simulink model "MPC_JUB27_galdir"  (R2021b)
settings: Solver=FixedStepDiscrete  StartTime=0.0  StopTime=StopTime  FixedStep=Ts  MaxStep=0.01  RelTol=1e-3
values from neighbouring files (symbols this model uses):
  dumax = [0.1 , 1]    [CarregaDados.m]    (also in Copy_of_casadi_block_Control.m = evalin('base','dumax'); casadi_block_Control.m = evalin('base','dumax'))
  f_buscaLimites_sym = evalin('base', 'f_buscaLimites_sym')    [Copy_of_casadi_block_Control.m]    (also in casadi_block_Control.m; casadi_block_Control_file.m; casadi_block_Control_galdir.m; casadi_block_Control_gov_ref.m)
  FreqAlvoIni = 55    [CarregaDados.m]
  Hc = Hp    (= 3)    [CarregaDadosMPC.m]    (also in Copy_of_casadi_block_Control.m = obj.Hc; casadi_block_Control.m = obj.Hc; casadi_block_Control_file.m = evalin('base','Hc');   obj.Hc=Hc; casadi_block_Control_galdir.m = obj.Hc)
  Hp = 3    [CarregaDadosMPC.m]    (also in Copy_of_casadi_block_Control.m = obj.Hp; casadi_block_Control.m = obj.Hp; casadi_block_Control_file.m = evalin('base','Hp');  obj.Hp=Hp; casadi_block_Control_galdir.m = obj.Hp)
  LimiteProporcao = Ts/TempoESN    (= 641.025641026)    [CarregaDados.m]
  MargemPercentual = 1    [CarregaDados.m]    (also in Copy_of_casadi_block_Control.m = evalin('base','MargemPercentual'); casadi_block_Control.m = evalin('base','MargemPercentual'))
  matriz_h = zeros(2,height(XIni))    [CarregaDados.m]    (also in Copy_of_casadi_block_Control.m = evalin('base','matriz_h'); casadi_block_Control.m = evalin('base','matriz_h'); casadi_block_Control_file.m = evalin('base','matriz_h'); casadi_block_Control_galdir.m = evalin('base','matriz_h'))
  nu = length(Qu)    [CarregaDadosMPC.m]    (also in Copy_of_casadi_block_Control.m = obj.nu; calc_ESNx_x_u.m = length(UIni); casadi_block_Control.m = obj.nu; casadi_block_Control_file.m = height(Qu))
  NumCasasDecimais = 1    [CarregaDados.m]
  nx = length(Qx)    [CarregaDadosMPC.m]    (also in Copy_of_casadi_block_Control.m = obj.nx; calc_ESN_controle.m = 10; calc_ESNx_x_u.m = height(YIni); casadi_block_Control.m = obj.nx)
  ny = length(Qy)    [CarregaDadosMPC.m]    (also in Copy_of_casadi_block_Control.m = obj.ny; casadi_block_Control.m = obj.ny; casadi_block_Control_file.m = height(Qy); casadi_block_Control_galdir.m = obj.ny)
  PassoMPC = 3    [CarregaDadosMPC.m]    (also in Copy_of_casadi_block_Control.m = obj.PassoMPC; casadi_block_Control.m = obj.PassoMPC; casadi_block_Control_file.m = evalin('base','PassoMPC'); casadi_block_Control_galdir.m = obj.PassoMPC)
  Plano = readtable('PlanoAceleracaoErro.xlsx')    [CarregaDados.m]
  PMonAlvoIni = max([PMonAlvoIni, Limites(2,2),PMonAlvoMaxMin(2)])    [CarregaDados.m]
  PMonAlvoMaxMin = [50 , 20]    [CarregaDados.m]
  Rede_Processo = load('weightsESNx_TR300_TVaz0.8_RaioE0.1.mat')    [CarregaDados.m]
  SNR = 20    [CarregaDados.m]
  Ts = 10    [CarregaDados.m]    (also in IncializaSolver.m = ModeloLSTM.temperatura_succao_BCSS.modelo_casadi.casadi_func; IncializaSolver_v2.m = ModeloLSTM.temperatura_succao_BCSS.modelo_casadi.casadi_func)
  UIni = evalin('base','UIni')    [Copy_of_casadi_block_Control.m]    (also in casadi_block_Control.m; casadi_block_Control_file.m; casadi_block_Control_galdir.m; casadi_block_Control_gov_ref.m)
  umax = [FreqMaxMin(1) ,  PMonAlvoMaxMin(1)]    [CarregaDados.m]    (also in Copy_of_casadi_block_Control.m = evalin('base','umax'); casadi_block_Control.m = evalin('base','umax'))
  umin = [FreqMaxMin(2), PMonAlvoMaxMin(2)]    [CarregaDados.m]    (also in Copy_of_casadi_block_Control.m = evalin('base','umin'); casadi_block_Control.m = evalin('base','umin'))
  UsaPlano = 0    [CarregaDados.m]
  XIni = evalin('base','XIni')    [Copy_of_casadi_block_Control.m]    (also in casadi_block_Control.m; casadi_block_Control_file.m; casadi_block_Control_galdir.m; casadi_block_Control_gov_ref.m)
undefined symbols (not defined in the file or in its folder): awgn, BTP, MatrizSimulador, MatrizSimuladorContas, TabelaIsometricas, VerHistorico
libraries: simulink x1
settings Model: Creator=odilo  LastModifiedBy=galdir
settings SolverCC: AlgebraicLoopSolver=LineSearch
settings DebuggingCC: InheritedTsInSrcMsg=none  SFMachineParentedDataDiag=warning

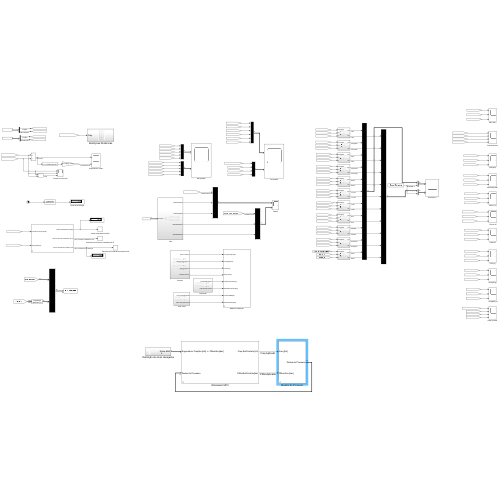
[thumbnail: Simulink's stored preview of the top-level diagram]
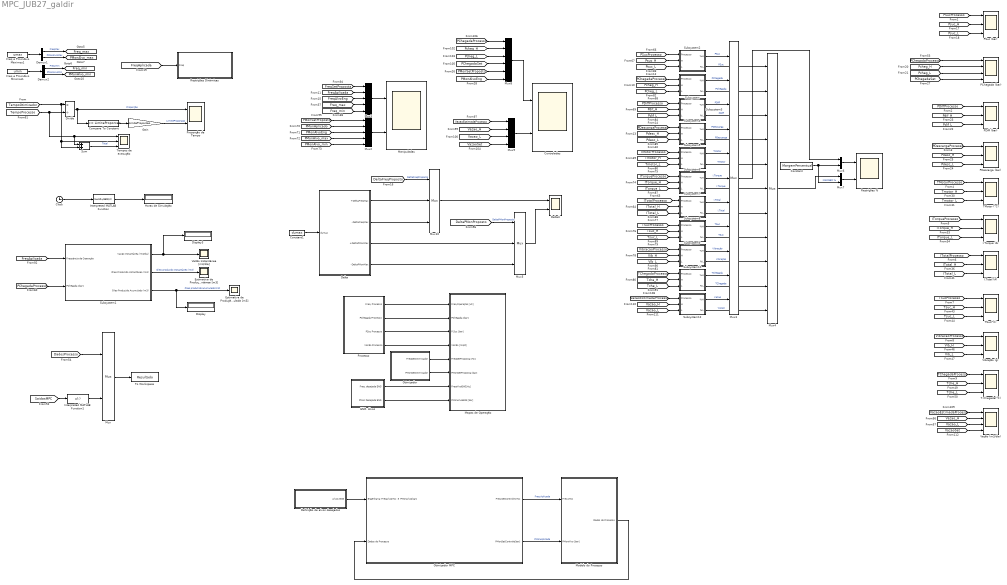
== system MPC_JUB27_galdir ==
  Clock : Clock
  Compare To Constant : simulink/Logic and Bit Operations/Compare To Constant  relop=<=  const=LimiteProporcao  OutDataTypeStr=boolean
  Constant : Constant  Value=MargemPercentual
  Constant1 : Constant  Value=dumax
  Controladas : Scope  NumInputPorts=2
  Definição de alvos desejados : Subsystem
  Delta : Subsystem
  DeltaU : Scope  NumInputPorts=2
  Demux1 : Demux  Outputs=2
  Demux2 : Demux  Outputs=2
  Display : Display
  Display3 : Display
  Divide : Product  Inputs=*/
  ENG. Alvos : Subsystem
  Estimativa de Produção Acumulada [m3] : Scope
  Estimativa de Produção instantânea [m3] : Scope
  Freq e PmonAlvo Máximos1 : Constant  Value=umax
  Freq e PmonAlvo Mínimos1 : Constant  Value=umin
  Gain : Gain  Gain=LimiteProporcao
  Horas de Simulação : Display
  I.Torque (A) : Scope  NumInputPorts=3
  I.Total (A) : Scope  NumInputPorts=3
  Interpreted MATLAB Function : MATLABFcn  MATLABFcn=round(u/3600,2)
  Interpreted MATLAB Function1 : MATLABFcn  MATLABFcn=u(:)
  Manipuladas : Scope  NumInputPorts=2
  Mapas de Operação : Subsystem  mask{PlotaMapas=1, HabilitaRastro=1, MatrizSimulador=MatrizSimulador, MatrizSimuladorContas=MatrizSimuladorContas, BTP=BTP, TabelaIsometricas=TabelaIsometricas, FreqIni=UIni(1), PChegadaIni=XIni(2), PSucIni=XIni(1), VazaoIni=XIni(11), MargemPercentual=MargemPercentual, FreqAlvoIni=FreqAlvoIni, PMonAlvoIni=PMonAlvoIni, PMonAlvoMaxMin=PMonAlvoMaxMin}
      mask prompts: PlotaMapas "Plotar Mapas (1/0)?"; HabilitaRastro "Habilita Rastro do Plot (1/0)?"; MatrizSimulador "Matriz do Simulador"; MatrizSimuladorContas "Matriz do Simulador para Limites"; BTP "Matriz BTP"; TabelaIsometricas "Tabela Curvas Isometricas"; FreqIni "Frequencia Inicial [Hz]"; PChegadaIni "PChegada Inicial [bar]"; PSucIni "PSuc Inicial [bar]"; VazaoIni "Vazao Inicial [m3/d]"; MargemPercentual "Margem % de folga para os alarmes"; FreqAlvoIni "Frequencia ALVO Inicial [Hz]"; PMonAlvoIni "PChegada ALVO [bar]"; PMonAlvoMaxMin "PMonAlvo [Max  Min]"
      mask DialogControl DescTextVar Prompt: MAPAS DE OPERAÇÃO
      mask DialogControl ParameterGroupVar Prompt: Tabelas Petrobras e configurações dos Mapas de Operação
      mask DialogControl ParameterGroupVar_copy Prompt: Dados do Processo
      mask DialogControl ParameterGroupVar_copy_copy_copy Prompt: Dados Engenharia (Alvos)
  Modelo do Processo : Subsystem  mask{ESN=Rede_Processo, YIni=XIni, UIni=UIni, SNR=SNR, NumCasasDecimais=NumCasasDecimais, MatrizSimulador=MatrizSimulador}
      mask prompts: ESN "Estruturada ESN"; YIni "Condicoes iniciais das variaveis"; UIni "Condicao Inicial das manipuladas (Freq e PMon)"; SNR "Relação Sinal Ruido aplicada"; NumCasasDecimais "Numero de casas decimais"; MatrizSimulador "Matriz do Simulador Petrobras"
  Mux : Mux  Inputs=2
  Mux1 : Mux  Inputs=5
  Mux10 : Mux  Inputs=3
  Mux2 : Mux  Inputs=5
  Mux3 : Mux  Inputs=11
  Mux4 : Mux  Inputs=11
  Mux5 : Mux  Inputs=3
  Mux6 : Mux  Inputs=2
  Mux7 : Mux  Inputs=2
  Mux8 : Mux  Inputs=6
  Mux9 : Mux
  Otimizador : Subsystem
  Otimizador MPC : Subsystem  mask{Hp=Hp, Hc=Hc, PassoMPC=PassoMPC, nx=nx, ny=ny, nu=nu}
      mask prompts: Hp "Horizonte de Predicao"; Hc "Horizonte de Controle"; PassoMPC "Passos para o controle atuar"; nx "Numero de Estados X"; ny "Numero de Saidas Y (controladas por setpoint)"; nu "Numero de entradas (acoes de controle)"
      mask DialogControl ControlParameters Prompt: PARAMETROS DO CONTROLADOR
      mask DialogControl SaidasCasadi Prompt: DIMENSIONAR SAIDAS CasadiBlock
  PChegada (bar) : Scope  NumInputPorts=4
  PDescarga (bar) : Scope  NumInputPorts=3
  PDiff (bar) : Scope  NumInputPorts=3
  PSuc (bar) : Scope  NumInputPorts=3
  Processo : Subsystem
  Proporção de Tempo : Scope  NumInputPorts=2
  Restrições % : Scope  NumInputPorts=2
  Restrições Dinâmicas : Subsystem
  Subsystem : Subsystem
  Subsystem1 : Subsystem  mask{MatrizSimulador=MatrizSimulador, DeltaT=Ts, QIni=XIni(11)}
      mask prompts: MatrizSimulador "Matriz do Simulador Petrobras"; DeltaT "Periodo de amostragem (s)"; QIni "Vazao Inicial (m3/dia)"
  Subsystem10 : Subsystem
  Subsystem12 : Subsystem
  Subsystem2 : Subsystem
  Subsystem3 : Subsystem
  Subsystem4 : Subsystem
  Subsystem5 : Subsystem
  Subsystem6 : Subsystem
  Subsystem7 : Subsystem
  Subsystem8 : Subsystem
  Subsystem9 : Subsystem
  Sum : Sum
  T.Chegada(°C) : Scope  NumInputPorts=3
  TMotor (°C) : Scope  NumInputPorts=3
  TSuc(°C) : Scope  NumInputPorts=3
  Tempos de execução : Scope  NumInputPorts=3
  To Workspace : ToWorkspace  VariableName=Resultado  SampleTime=-1
  Vazão (m3/dia) : Scope  NumInputPorts=4
  Vazão Instantânea [m3/dia] : Scope
  Vibração (g) : Scope  NumInputPorts=3
  tag scope: Freq_max=global, Freq_min=global, PMonAlvo_max=global, PMonAlvo_min=global
  wires:
  [TempoProcesso] -> Sum/1, Tempos de execução/1, Divide/2
  [ITotalProcesso] -> I.Total (A)/1
  [TMotorProcesso] -> TMotor (°C)/1
  [VibracaoProcesso] -> Vibração (g)/1
  [TSucProcesso] -> TSuc(°C)/1
  [PDiffProcesso] -> PDiff (bar)/1
  [PDescargaProcesso] -> PDescarga (bar)/1
  [PSucProcesso] -> PSuc (bar)/1
  [Freq_max] -> Mux1/4
  [Freq_min] -> Mux1/5
  [FreqAlvoEng] -> Mux1/3
  [Psuc_H] -> PSuc (bar)/2
  [Psuc_L] -> PSuc (bar)/3
  [Pdif_H] -> PDiff (bar)/2
  [Pdif_L] -> PDiff (bar)/3
  [Pdesc_H] -> PDescarga (bar)/2
  [Pdesc_L] -> PDescarga (bar)/3
  [Tmotor_H] -> TMotor (°C)/2
  [Tmotor_L] -> TMotor (°C)/3
  [ITorqueProcesso] -> I.Torque (A)/1
  [ITorque_H] -> I.Torque (A)/2
  [ITorque_L] -> I.Torque (A)/3
  [ITotal_H] -> I.Total (A)/2
  [ITotal_L] -> I.Total (A)/3
  [Tsuc_H] -> TSuc(°C)/2
  [Tsuc_L] -> TSuc(°C)/3
  [Vib_H] -> Vibração (g)/2
  [Vib_L] -> Vibração (g)/3
  [TChegadaProcesso] -> T.Chegada(°C)/1
  [Tche_H] -> T.Chegada(°C)/2
  [Tche_L] -> T.Chegada(°C)/3
  Mux/1 -> To Workspace/1
  [DadosProcesso] -> Mux/1
  [FreqAplicada] -> Mux1/2
  [PChegadaProcesso] -> PChegada (bar)/1
  [Pcheg_H] -> PChegada (bar)/2
  [Pcheg_L] -> PChegada (bar)/3
  [PChegadaSet] -> PChegada (bar)/4
  [TempoOtimizador] -> Sum/2, Tempos de execução/2, Divide/1
  [FreqAplicada] -> Subsystem1/1(Frequência de Operação)
  [PChegadaProcesso] -> Subsystem1/2(PChegada [bar])
  Subsystem1/2("Óleo Produzido Instantâneo (m3) ") -> Estimativa de Produção instantânea [m3]/1  "Óleo produzido Instantâneo (m3)"
  Subsystem1/3(Óleo Produzido Acumulado (m3)) -> Display/1, Estimativa de Produção Acumulada [m3]/1  "Óleo produzido acumulado(m3)"
  Subsystem1/1(Vazão Instantânea (m3/dia)) -> Display3/1, Vazão Instantânea [m3/dia]/1
  Sum/1 -> Tempos de execução/3  "Total"
  Mux1/1 -> Manipuladas/1
  [PMonAlvo_min] -> Mux2/5
  [PMonAlvo_max] -> Mux2/4
  [PMonAplicado] -> Mux2/2
  Mux2/1 -> Manipuladas/2
  [PChegadaProcesso] -> Subsystem/1(Processo)
  [Pcheg_H] -> Subsystem/2(H)
  [Pcheg_L] -> Subsystem/3(L)
  [PSucProcesso] -> Subsystem2/1(Processo)
  [Psuc_H] -> Subsystem2/2(H)
  [Psuc_L] -> Subsystem2/3(L)
  [PDiffProcesso] -> Subsystem3/1(Processo)
  [Pdif_H] -> Subsystem3/2(H)
  [Pdif_L] -> Subsystem3/3(L)
  [PDescargaProcesso] -> Subsystem4/1(Processo)
  [Pdesc_H] -> Subsystem4/2(H)
  [Pdesc_L] -> Subsystem4/3(L)
  [Tmotor_L] -> Subsystem5/3(L)
  [Tmotor_H] -> Subsystem5/2(H)
  [TMotorProcesso] -> Subsystem5/1(Processo)
  [ITorqueProcesso] -> Subsystem6/1(Processo)
  [ITorque_H] -> Subsystem6/2(H)
  [ITorque_L] -> Subsystem6/3(L)
  [ITotalProcesso] -> Subsystem7/1(Processo)
  [ITotal_H] -> Subsystem7/2(H)
  [ITotal_L] -> Subsystem7/3(L)
  [TSucProcesso] -> Subsystem8/1(Processo)
  [Tsuc_H] -> Subsystem8/2(H)
  [Tsuc_L] -> Subsystem8/3(L)
  [VibracaoProcesso] -> Subsystem9/1(Processo)
  [Vib_H] -> Subsystem9/2(H)
  [Vib_L] -> Subsystem9/3(L)
  [TChegadaProcesso] -> Subsystem10/1(Processo)
  [Tche_H] -> Subsystem10/2(H)
  [Tche_L] -> Subsystem10/3(L)
  Mux3/1 -> Mux6/1
  Mux4/1 -> Mux7/1
  Subsystem/2(%L) -> Mux4/2  "PChegada"
  Subsystem2/2(%L) -> Mux4/1  "PSuc"
  Subsystem/1(%H) -> Mux3/2  "PChegada"
  Subsystem2/1(%H) -> Mux3/1  "PSuc"
  Subsystem3/1(%H) -> Mux3/3  "PDiff"
  Subsystem3/2(%L) -> Mux4/3  "PDiff"
  Subsystem4/1(%H) -> Mux3/4  "PDescarga"
  Subsystem4/2(%L) -> Mux4/4  "PDescarga"
  Subsystem5/2(%L) -> Mux4/5  "TMotor"
  Subsystem5/1(%H) -> Mux3/5  "TMotor"
  Subsystem6/2(%L) -> Mux4/6  "I.Torque"
  Subsystem6/1(%H) -> Mux3/6  "I.Torque"
  Subsystem7/2(%L) -> Mux4/7  "I.Total"
  Subsystem7/1(%H) -> Mux3/7  "I.Total"
  Subsystem8/2(%L) -> Mux4/8  "TSuc"
  Subsystem8/1(%H) -> Mux3/8  "TSuc"
  Subsystem9/2(%L) -> Mux4/9  "Vibração"
  Mux10/1 -> DeltaU/1
  Constant1/1 -> Delta/1(dumax)
  Delta/2(-DeltaFreqMax) -> Mux10/3
  Clock/1 -> Interpreted MATLAB Function/1
  Interpreted MATLAB Function/1 -> Horas de Simulação/1
  [DeltaPMonProposto] -> Mux5/1  "DeltaPMonProposto"
  Delta/3(+DeltaPMonMax) -> Mux5/2
  Delta/4(-DeltaPMonMax) -> Mux5/3
  [PChegadaSet] -> Mux8/4
  [Pcheg_L] -> Mux8/3
  [Pcheg_H] -> Mux8/2
  [PChegadaProcesso] -> Mux8/1
  [VazaoSet] -> Mux9/4
  [Vazao_L] -> Mux9/3
  [Vazao_H] -> Mux9/2
  [VazaoEstimadaProcesso] -> Mux9/1
  Mux9/1 -> Controladas/2
  Mux8/1 -> Controladas/1
  Processo/1(Freq. Processo) -> Mapas de Operação/1(Freq.Operação [Hz])
  Processo/2(PChegada Processo) -> Mapas de Operação/2(PChegada [bar])
  ENG. Alvos/1(Freq. desejada ENG) -> Mapas de Operação/7(FreqAlvoENG[Hz])
  ENG. Alvos/2(PMon Desejada ENG) -> Mapas de Operação/8(PMonAlvoENG [bar])
  Processo/3(PSuc Processo) -> Mapas de Operação/3(P.Suc [bar])
  Delta/1(+DeltaFreqMax) -> Mux10/2
  Otimizador MPC/1(Freq.SetControle [Hz]) -> Modelo do Processo/1(Freq [Hz])  "Freq.Aplicada"
  Otimizador MPC/2(PMonSetControle[bar]) -> Modelo do Processo/2(PMonAlvo [bar])  "PMonAplicada"
  [FreqSetProposta] -> Mux1/1
  [PMonSetProposto] -> Mux2/1
  [PMonAlvoEng] -> Mux2/3
  [Vazao_L] -> Vazão (m3/dia)/3
  [Vazao_H] -> Vazão (m3/dia)/2
  [VazaoEstimadaProcesso] -> Vazão (m3/dia)/1
  [VazaoEstimadaProcesso] -> Subsystem12/1(Processo)
  [Vazao_H] -> Subsystem12/2(H)
  [Vazao_L] -> Subsystem12/3(L)
  Subsystem12/1(%H) -> Mux3/11  "Vazao"
  Subsystem12/2(%L) -> Mux4/11  "Vazao"
  Subsystem10/2(%L) -> Mux4/10  "TChegada"
  Subsystem9/1(%H) -> Mux3/9  "Vibração"
  Subsystem10/1(%H) -> Mux3/10  "TChegada"
  [VazaoSet] -> Vazão (m3/dia)/4
  Modelo do Processo/1(Dados do Processo) -> Otimizador MPC/2(Dados do Processo)
  Divide/1 -> Proporção de Tempo/1, Compare To Constant/1  "Proporção"
  Compare To Constant/1 -> Gain/1
  Gain/1 -> Proporção de Tempo/2  "LimiteProporção"
  Definição de alvos desejados/1(Alvos ENG) -> Otimizador MPC/1(Engenharia: FreqAlvo[Hz]  e  PMonAlvo[bar])
  Demux1/1 -> [Freq_max]  "FreqMax"
  Demux2/1 -> [Freq_min]  "Freq.Min"
  Demux1/2 -> [PMonAlvo_max]  "PMonAlvoMax"
  Demux2/2 -> [PMonAlvo_min]  "PMonAlvoMin"
  Freq e PmonAlvo Mínimos1/1 -> Demux2/1
  Freq e PmonAlvo Máximos1/1 -> Demux1/1
  [FreqAplicada] -> Restrições Dinâmicas/1(Freq)
  Processo/4(Vazão Processo) -> Mapas de Operação/4(Vazão [m3/d])
  Otimizador/1(FreqSetOtimizador) -> Mapas de Operação/5(FreqSetProposta [Hz])
  Otimizador/2(PMonSetOtimizador) -> Mapas de Operação/6(PMonSetProposta [bar])
  [DeltaFreqProposto] -> Mux10/1  "DeltaFreqProposto"
  Mux5/1 -> DeltaU/2
  [PMonSetProposto] -> Mux8/5
  [PMonAlvoEng] -> Mux8/6
  Mux6/1 -> Restrições %/1
  Constant/1 -> Mux6/2, Mux7/2  "MARGEM %"
  Mux7/1 -> Restrições %/2
  [SaidasMPC] -> Interpreted MATLAB Function1/1
  Interpreted MATLAB Function1/1 -> Mux/2

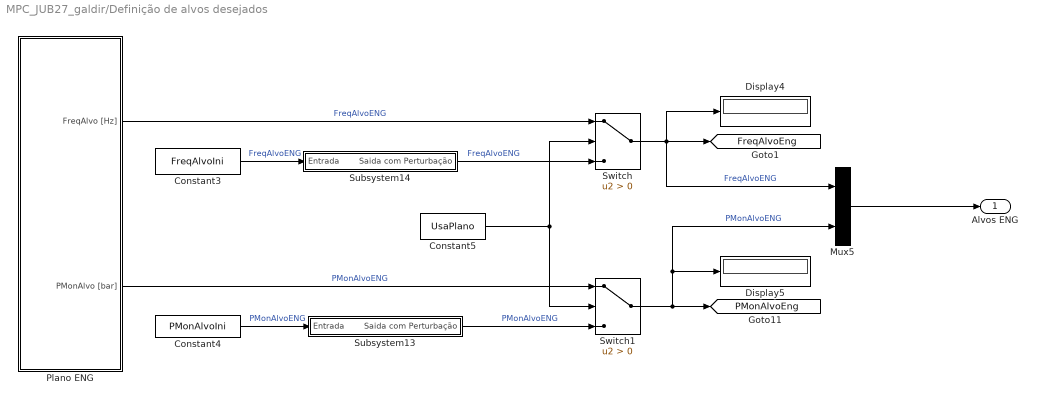
== system MPC_JUB27_galdir/Definição de alvos desejados ==
  Constant3 : Constant  Value=FreqAlvoIni
  Constant4 : Constant  Value=PMonAlvoIni
  Constant5 : Constant  Value=UsaPlano
  Display4 : Display
  Display5 : Display
  Mux5 : Mux  Inputs=2
  Plano ENG : Subsystem  mask{Plano=Plano}
      mask prompts: Plano "Plano de Execucao"
      mask DialogControl DescGroupVar Prompt: TABELA COM PLANO DE EXECUCAO
  Subsystem13 : Subsystem  mask{TIni=1200, DeltaT=1.5*3600, ValorP=0}
      mask prompts: TIni "Tempo Inicio"; DeltaT "Duracao"; ValorP "Valor da Perturbacao"
  Subsystem14 : Subsystem  mask{TIni=1200, DeltaT=1.5*3600, ValorP=0}
      mask prompts: TIni "Tempo Inicio"; DeltaT "Duracao"; ValorP "Valor da Perturbacao"
  Switch : Switch  Criteria=u2 > Threshold
  Switch1 : Switch  Criteria=u2 > Threshold
  Alvos ENG : Outport
  tag scope: FreqAlvoEng=global, PMonAlvoEng=global
  wires:
  Constant5/1 -> Switch1/2, Switch/2
  Subsystem14/1(Saida com Perturbação) -> Switch/3  "FreqAlvoENG"
  Constant3/1 -> Subsystem14/1(Entrada)  "FreqAlvoENG"
  Switch/1 -> Mux5/1, [FreqAlvoEng], Display4/1  "FreqAlvoENG"
  Switch1/1 -> Mux5/2, Display5/1, [PMonAlvoEng]  "PMonAlvoENG"
  Plano ENG/1(FreqAlvo [Hz]) -> Switch/1  "FreqAlvoENG"
  Subsystem13/1(Saida com Perturbação) -> Switch1/3  "PMonAlvoENG"
  Plano ENG/2(PMonAlvo [bar]) -> Switch1/1  "PMonAlvoENG"
  Constant4/1 -> Subsystem13/1(Entrada)  "PMonAlvoENG"
  Mux5/1 -> Alvos ENG/1

== system MPC_JUB27_galdir/Delta ==
  dumax : Inport
  Demux : Demux  Outputs=2
  Gain : Gain  Gain=-1
  Gain6 : Gain  Gain=-1
  +DeltaFreqMax : Outport
  -DeltaFreqMax : Outport  Port=2
  +DeltaPMonMax : Outport  Port=3
  -DeltaPMonMax : Outport  Port=4
  wires:
  Demux/1 -> Gain/1, +DeltaFreqMax/1  "+DeltaFreqMax"
  Demux/2 -> Gain6/1, +DeltaPMonMax/1  "+DeltaPMonMax"
  dumax/1 -> Demux/1
  Gain/1 -> -DeltaFreqMax/1  "-DeltaFreqMax"
  Gain6/1 -> -DeltaPMonMax/1  "-DeltaPMonMax"

== system MPC_JUB27_galdir/ENG. Alvos ==
  Freq. desejada ENG : Outport
  PMon Desejada ENG : Outport  Port=2
  wires:
  [PMonAlvoEng] -> PMon Desejada ENG/1
  [FreqAlvoEng] -> Freq. desejada ENG/1

== system MPC_JUB27_galdir/Mapas de Operação ==
  Freq.Operação [Hz] : Inport
  PChegada [bar] : Inport  Port=2
  P.Suc [bar] : Inport  Port=3
  Vazão [m3/d] : Inport  Port=4
  FreqSetProposta [Hz] : Inport  Port=5
  PMonSetProposta [bar] : Inport  Port=6
  FreqAlvoENG[Hz] : Inport  Port=7
  PMonAlvoENG [bar] : Inport  Port=8
  Mux : Mux  Inputs=8
  S-Function : S-Function  FunctionName=AnimaMapa  Parameters=PlotaMapas,MatrizSimulador,MatrizSimuladorContas,BTP,FreqIni, PChegadaIni,PSucIni,VazaoIni,FreqAlvoIni,PMonAlvoIni,HabilitaRastro,TabelaIsometricas,MargemPercentual,PMonAlvoMaxMin  SFunctionDeploymentMode=off  EnableBusSupport=off
  wires:
  FreqSetProposta [Hz]/1 -> Mux/5
  PMonAlvoENG [bar]/1 -> Mux/8
  FreqAlvoENG[Hz]/1 -> Mux/7
  PMonSetProposta [bar]/1 -> Mux/6
  Vazão [m3/d]/1 -> Mux/4
  PChegada [bar]/1 -> Mux/2
  Mux/1 -> S-Function/1
  Freq.Operação [Hz]/1 -> Mux/1
  P.Suc [bar]/1 -> Mux/3

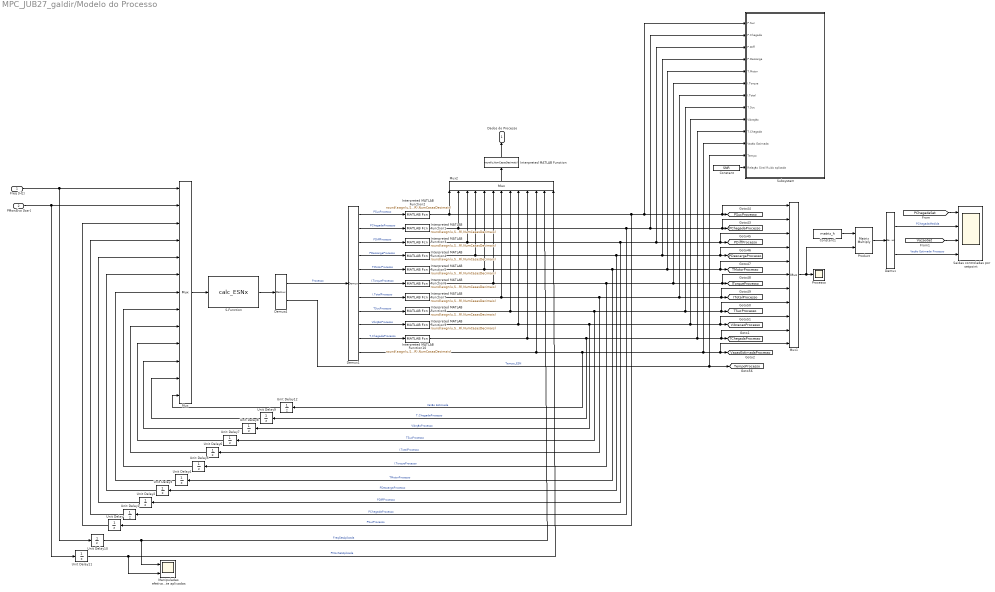
== system MPC_JUB27_galdir/Modelo do Processo ==
  Freq [Hz] : Inport
  PMonAlvo [bar] : Inport  Port=2
  Constant : Constant  Value=SNR
  Constant1 : Constant  Value=matriz_h
  Demux : Demux  Outputs=2
  Demux1 : Demux  Outputs=11
  Demux4 : Demux  Outputs=[ 11 1]
  Interpreted MATLAB Function : MATLABFcn  MATLABFcn=round(u,NumCasasDecimais)
  Interpreted MATLAB Function{1..10} (10 alike) : MATLABFcn  MATLABFcn=round(awgn(u,SNR),NumCasasDecimais)
  Manipuladas efetivamente aplicadas : Scope  NumInputPorts=2
  Mux : Mux  Inputs=2+11
  Mux1 : Mux  Inputs=11
  Mux2 : Mux  Inputs=13
  Processo : Scope
  Product : Product  Multiplication=Matrix(*)
  S-Function : S-Function  FunctionName=calc_ESNx  Parameters=ESN.data,YIni,MatrizSimulador  SFunctionDeploymentMode=off  EnableBusSupport=off
  Saidas controladas por setpoint : Scope  NumInputPorts=4
  Subsystem : Subsystem
  Unit Delay : UnitDelay  InitialCondition=YIni(1)  SampleTime=-1  HasFrameUpgradeWarning=on
  Unit Delay1 : UnitDelay  InitialCondition=YIni(2)  SampleTime=-1  HasFrameUpgradeWarning=on
  Unit Delay10 : UnitDelay  InitialCondition=UIni(1)  SampleTime=-1  HasFrameUpgradeWarning=on
  Unit Delay11 : UnitDelay  InitialCondition=UIni(2)  SampleTime=-1  HasFrameUpgradeWarning=on
  Unit Delay12 : UnitDelay  InitialCondition=YIni(11)  SampleTime=-1  HasFrameUpgradeWarning=on
  Unit Delay2 : UnitDelay  InitialCondition=YIni(3)  SampleTime=-1  HasFrameUpgradeWarning=on
  Unit Delay3 : UnitDelay  InitialCondition=YIni(4)  SampleTime=-1  HasFrameUpgradeWarning=on
  Unit Delay4 : UnitDelay  InitialCondition=YIni(5)  SampleTime=-1  HasFrameUpgradeWarning=on
  Unit Delay5 : UnitDelay  InitialCondition=YIni(6)  SampleTime=-1  HasFrameUpgradeWarning=on
  Unit Delay6 : UnitDelay  InitialCondition=YIni(7)  SampleTime=-1  HasFrameUpgradeWarning=on
  Unit Delay7 : UnitDelay  InitialCondition=YIni(8)  SampleTime=-1  HasFrameUpgradeWarning=on
  Unit Delay8 : UnitDelay  InitialCondition=YIni(9)  SampleTime=-1  HasFrameUpgradeWarning=on
  Unit Delay9 : UnitDelay  InitialCondition=YIni(10)  SampleTime=-1  HasFrameUpgradeWarning=on
  Dados do Processo : Outport
  tag scope: ITorqueProcesso=global, ITotalProcesso=global, PChegadaProcesso=global, PDescargaProcesso=global, PDiffProcesso=global, PSucProcesso=global, TChegadaProcesso=global, TMotorProcesso=global, TSucProcesso=global, TempoProcesso=global, VazaoEstimadaProcesso=global, VibracaoProcesso=global
  wires:
  Mux/1 -> S-Function/1
  PMonAlvo [bar]/1 -> Unit Delay11/1, Mux/2
  Freq [Hz]/1 -> Unit Delay10/1, Mux/1
  Unit Delay/1 -> Mux/3
  Unit Delay1/1 -> Mux/4
  Unit Delay2/1 -> Mux/5
  Unit Delay3/1 -> Mux/6
  Unit Delay4/1 -> Mux/7
  Unit Delay5/1 -> Mux/8
  Unit Delay6/1 -> Mux/9
  Unit Delay7/1 -> Mux/10
  Unit Delay8/1 -> Mux/11
  Unit Delay9/1 -> Mux/12
  S-Function/1 -> Demux4/1
  Demux1/4 -> Interpreted MATLAB Function4/1  "PDescargaProcesso"
  Demux1/3 -> Interpreted MATLAB Function3/1  "PDiffProcesso"
  Demux1/9 -> Interpreted MATLAB Function9/1  "VibrçãoProcesso"
  Demux1/7 -> Interpreted MATLAB Function7/1  "I.TotalProcesso"
  Demux1/10 -> Interpreted MATLAB Function10/1  "T,ChegadaProcesso"
  Demux4/2 -> Subsystem/12(Tempo), [TempoProcesso]  "Tempo_ESN"
  Interpreted MATLAB Function2/1 -> Unit Delay/1, Subsystem/1(P.Suc), Mux1/1, [PSucProcesso], Mux2/1  "PSucProcesso"
  Interpreted MATLAB Function1/1 -> Subsystem/2(P.Chegada), Mux1/2, [PChegadaProcesso], Unit Delay1/1, Mux2/2  "PChegadaProcesso"
  Interpreted MATLAB Function3/1 -> Subsystem/3(P.Diff), Mux1/3, [PDiffProcesso], Unit Delay2/1, Mux2/3  "PDiffProcesso"
  Interpreted MATLAB Function4/1 -> Subsystem/4(P.Descarga), Mux1/4, [PDescargaProcesso], Unit Delay3/1, Mux2/4  "PDescargaProcesso"
  Interpreted MATLAB Function5/1 -> Subsystem/5(T.Motor), Mux1/5, [TMotorProcesso], Unit Delay4/1, Mux2/5  "TMotorProcesso"
  Interpreted MATLAB Function6/1 -> Subsystem/6(I.Torque), Mux1/6, [ITorqueProcesso], Unit Delay5/1, Mux2/6  "I.TorqueProcesso"
  Interpreted MATLAB Function7/1 -> Subsystem/7(I.Total), Mux1/7, [ITotalProcesso], Unit Delay6/1, Mux2/7  "I.TotalProcesso"
  Interpreted MATLAB Function8/1 -> Subsystem/8(T.Suc), Mux1/8, [TSucProcesso], Unit Delay7/1, Mux2/8  "TSucProcesso"
  Interpreted MATLAB Function9/1 -> Subsystem/9(Vibração), Mux1/9, [VibracaoProcesso], Unit Delay8/1, Mux2/9  "VibrçãoProcesso"
  Interpreted MATLAB Function10/1 -> Unit Delay9/1, Mux1/10, [TChegadaProcesso], Subsystem/10(T.Chegada), Mux2/10  "T,ChegadaProcesso"
  Constant/1 -> Subsystem/13(Relação Sinal Ruido aplicada)
  Demux1/1 -> Interpreted MATLAB Function2/1  "PSucProcesso"
  Demux1/2 -> Interpreted MATLAB Function1/1  "PChegadaProcesso"
  Demux1/5 -> Interpreted MATLAB Function5/1  "TMotorProcesso"
  Demux1/6 -> Interpreted MATLAB Function6/1  "I.TorqueProcesso"
  Demux1/8 -> Interpreted MATLAB Function8/1  "TSucProcesso"
  Interpreted MATLAB Function/1 -> Dados do Processo/1
  Demux4/1 -> Demux1/1  "Processo"
  Unit Delay10/1 -> Mux2/12, Manipuladas efetivamente aplicadas/1  "FreqSetAplicada"
  Unit Delay11/1 -> Mux2/13, Manipuladas efetivamente aplicadas/2  "PMonSetAplicada"
  Demux1/11 -> Subsystem/11(Vazão Estimada), Mux1/11, [VazaoEstimadaProcesso], Unit Delay12/1, Mux2/11  "Vazão Estimada"
  Unit Delay12/1 -> Mux/13
  Product/1 -> Demux/1
  Constant1/1 -> Product/1
  Mux1/1 -> Product/2, Processo/1
  [PChegadaSet] -> Saidas controladas por setpoint/1
  [VazaoSet] -> Saidas controladas por setpoint/3
  Demux/1 -> Saidas controladas por setpoint/2  "PChegadaMedida"
  Demux/2 -> Saidas controladas por setpoint/4  "Vazão Estimada Processo"
  Mux2/1 -> Interpreted MATLAB Function/1

== system MPC_JUB27_galdir/Otimizador ==
  FreqSetOtimizador : Outport
  PMonSetOtimizador : Outport  Port=2
  wires:
  [FreqSetProposta] -> FreqSetOtimizador/1
  [PMonSetProposto] -> PMonSetOtimizador/1

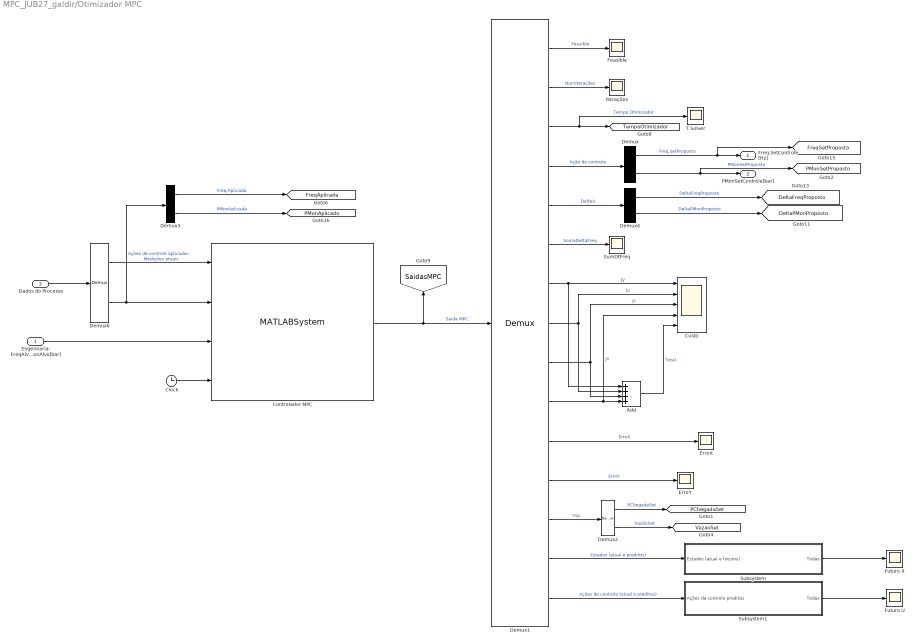
== system MPC_JUB27_galdir/Otimizador MPC ==
  Engenharia: FreqAlvo[Hz]  e  PMonAlvo[bar] : Inport
  Dados do Processo : Inport  Port=2
  Add : Sum  Inputs=++++
  Clock : Clock
  Controlador MPC : MATLABSystem  System=casadi_block_Control  SimulateUsing=Interpreted execution
      mask Type: casadi_block_Control
      mask Display:
      | disp('casadi_block_Control');
      | port_label('input',1,'X0');
      | port_label('input',2,'U0');
      | port_label('input',3,'AlvoEng');
      | port_label('input',4,'t');
      | port_label('output',1,'SaidaMPC');
  "Custo " : Scope  NumInputPorts=5
  Demux{,2..4} (4 alike) : Demux  Outputs=2
  Demux1 : Demux  Outputs="[ 1  1  1  nu  nu  1  1  1  1  1  nx  ny  ny    nx+nx*Hp   nu*Hp ]"
  Demux6 : Demux  Outputs=[11 2]
  ErroX : Scope
  ErroY : Scope
  Feasible : Scope
  Futuro U : Scope
  Futuro X : Scope
  Iterações : Scope
  Subsystem : Subsystem
  Subsystem1 : Subsystem
  SumDtFreq : Scope
  T.Solver : Scope
  Freq.SetControle [Hz] : Outport
  PMonSetControle[bar] : Outport  Port=2
  tag scope: DeltaFreqProposto=global, DeltaPMonProposto=global, FreqAplicada=global, FreqSetProposta=global, PChegadaSet=global, PMonAplicado=global, PMonSetProposto=global, SaidasMPC=global, TempoOtimizador=global, VazaoSet=global
  wires:
  Demux1/3 -> T.Solver/1, [TempoOtimizador]  "Tempo Otimizador"
  Demux1/1 -> Feasible/1  "Feasible"
  Demux4/1 -> [DeltaFreqProposto]  "DeltaFreqProposto"
  Demux/1 -> [FreqSetProposta], Freq.SetControle [Hz]/1  "Freq.SetProposto"
  Demux/2 -> [PMonSetProposto], PMonSetControle[bar]/1  "PMonSetProposto"
  Demux4/2 -> [DeltaPMonProposto]  "DeltaPMonProposto"
  Dados do Processo/1 -> Demux6/1
  Demux6/1 -> Controlador MPC/1  "Medições atuais"
  Demux6/2 -> Demux3/1, Controlador MPC/2  "Ações de controle aplicadas"
  Demux1/4 -> Demux/1  "Ação de controle"
  Demux1/2 -> Iterações/1  "NumIterações"
  Demux1/5 -> Demux4/1  "DeltaU"
  Controlador MPC/1 -> [SaidasMPC], Demux1/1  "Saida MPC"
  Demux2/1 -> [PChegadaSet]  "PChegadaSet"
  Engenharia: FreqAlvo[Hz]  e  PMonAlvo[bar]/1 -> Controlador MPC/3
  Demux2/2 -> [VazaoSet]  "VazãoSet"
  Clock/1 -> Controlador MPC/4
  Demux3/2 -> [PMonAplicado]  "PMonAplicada"
  Demux3/1 -> [FreqAplicada]  "Freq.Aplicada"
  Demux1/14 -> Subsystem/1(Estados (atual e futuros))  "Estados (atual e preditos)"
  Subsystem/1(Todas) -> Futuro X/1
  Subsystem1/1(Todas) -> Futuro U/1
  Demux1/6 -> SumDtFreq/1  "SomaDeltaFreq"
  Demux1/7 -> "Custo "/1, Add/1  "Jy"
  Demux1/8 -> "Custo "/2, Add/2  "Ju"
  Demux1/9 -> "Custo "/3, Add/3  "Jr"
  Demux1/13 -> Demux2/1  "Ysp"
  Demux1/10 -> "Custo "/4, Add/4  "Jx"
  Add/1 -> "Custo "/5  "Total"
  Demux1/15 -> Subsystem1/1(Ações de controle preditas)  "Ações de controle (atual e preditos)"
  Demux1/11 -> ErroX/1  "ErroX"
  Demux1/12 -> ErroY/1  "ErroY"

== system MPC_JUB27_galdir/Processo ==
  Freq. Processo : Outport
  PChegada Processo : Outport  Port=2
  PSuc Processo : Outport  Port=3
  Vazão Processo : Outport  Port=4
  wires:
  [PSucProcesso] -> PSuc Processo/1
  [FreqAplicada] -> Freq. Processo/1
  [PChegadaProcesso] -> PChegada Processo/1
  [VazaoEstimadaProcesso] -> Vazão Processo/1

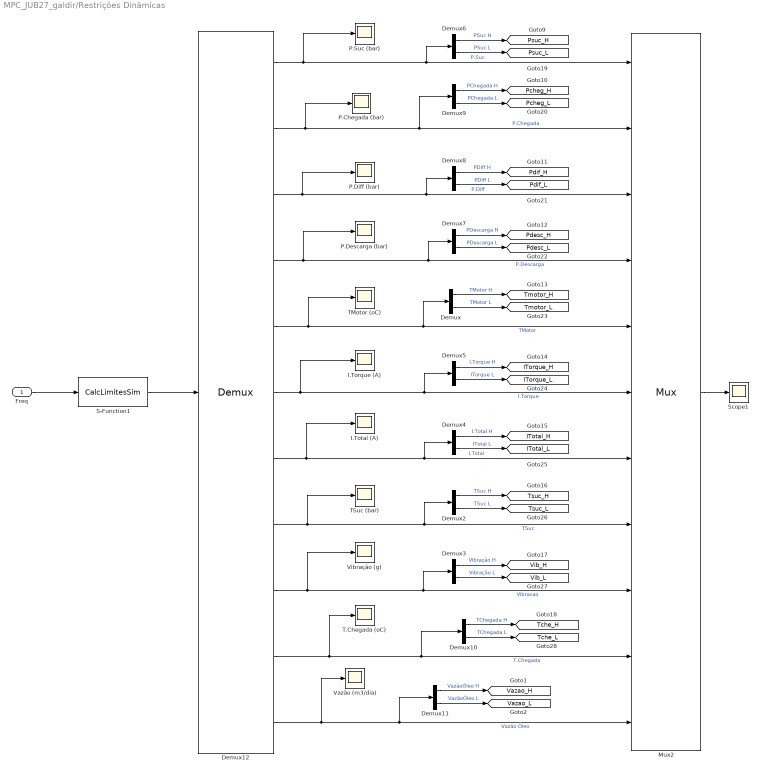
== system MPC_JUB27_galdir/Restrições Dinâmicas ==
  Freq : Inport
  Demux{,2..11} (11 alike) : Demux  Outputs=2
  Demux12 : Demux  Outputs=[ 2 2 2 2 2 2 2 2 2 2 2]
  I.Torque (A) : Scope
  I.Total (A) : Scope
  Mux2 : Mux  Inputs=[ 2 2 2 2 2 2 2 2 2 2 2]
  P.Chegada (bar) : Scope
  P.Descarga (bar) : Scope
  P.Diff (bar) : Scope
  P.Suc (bar) : Scope
  S-Function1 : S-Function  FunctionName=CalcLimitesSim  Parameters=UIni(1),f_buscaLimites_sym  SFunctionDeploymentMode=off  EnableBusSupport=off
  Scope1 : Scope
  T.Chegada (oC) : Scope
  TMotor (oC) : Scope
  TSuc (bar) : Scope
  Vazão (m3/dia) : Scope
  Vibração (g) : Scope
  tag scope: ITorque_H=global, ITorque_L=global, ITotal_H=global, ITotal_L=global, Pcheg_H=global, Pcheg_L=global, Pdesc_H=global, Pdesc_L=global, Pdif_H=global, Pdif_L=global, Psuc_H=global, Psuc_L=global, Tche_H=global, Tche_L=global, Tmotor_H=global, Tmotor_L=global, Tsuc_H=global, Tsuc_L=global, Vazao_H=global, Vazao_L=global, Vib_H=global, Vib_L=global
  wires:
  Demux12/9 -> Vibração (g)/1, Demux3/1, Mux2/9  "Vibracao"
  Demux12/4 -> P.Descarga (bar)/1, Demux7/1, Mux2/4  "P.Descarga"
  Demux12/10 -> T.Chegada (oC)/1, Demux10/1, Mux2/10  "T.Chegada"
  Demux12/1 -> P.Suc (bar)/1, Mux2/1, Demux6/1  "P.Suc"
  Demux12/2 -> P.Chegada (bar)/1, Demux9/1, Mux2/2  "P.Chegada"
  Demux12/3 -> P.Diff (bar)/1, Mux2/3, Demux8/1  "P.Diff"
  Demux12/5 -> TMotor (oC)/1, Demux/1, Mux2/5  "TMotor"
  Demux12/8 -> TSuc (bar)/1, Demux2/1, Mux2/8  "TSuc"
  Demux12/6 -> I.Torque (A)/1, Demux5/1, Mux2/6  "I.Torque"
  Demux12/7 -> I.Total (A)/1, Demux4/1, Mux2/7  "I.Total"
  Demux/2 -> [Tmotor_L]  "TMotor L"
  Demux/1 -> [Tmotor_H]  "TMotor H"
  Demux6/1 -> [Psuc_H]  "PSuc H"
  Demux9/1 -> [Pcheg_H]  "PChegada H"
  Demux8/1 -> [Pdif_H]  "PDiff H"
  Demux7/1 -> [Pdesc_H]  "PDescarga H"
  Demux5/1 -> [ITorque_H]  "I.Torque H"
  Demux4/1 -> [ITotal_H]  "I.Total H"
  Demux2/1 -> [Tsuc_H]  "TSuc H"
  Demux3/1 -> [Vib_H]  "Vibração H"
  Demux10/1 -> [Tche_H]  "TChegada H"
  Demux6/2 -> [Psuc_L]  "PSuc L"
  Demux9/2 -> [Pcheg_L]  "PChegada L"
  Demux8/2 -> [Pdif_L]  "PDiff L"
  Demux7/2 -> [Pdesc_L]  "PDescarga L"
  Demux4/2 -> [ITotal_L]  "ITotal L"
  Demux2/2 -> [Tsuc_L]  "TSuc L"
  Demux3/2 -> [Vib_L]  "Vibração L"
  Demux10/2 -> [Tche_L]  "TChegada L"
  Demux5/2 -> [ITorque_L]  "ITorque L"
  Demux12/11 -> Demux11/1, Mux2/11, Vazão (m3/dia)/1  "Vazão Óleo"
  Demux11/2 -> [Vazao_L]  "VazãoÓleo L"
  Demux11/1 -> [Vazao_H]  "VazãoÓleo H"
  S-Function1/1 -> Demux12/1
  Freq/1 -> S-Function1/1
  Mux2/1 -> Scope1/1

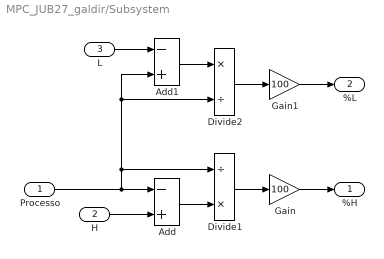
== system MPC_JUB27_galdir/Subsystem ==
  Processo : Inport
  H : Inport  Port=2
  L : Inport  Port=3
  Add : Sum  Inputs=-+
  Add1 : Sum  Inputs=-+
  Divide1 : Product  Inputs=/*
  Divide2 : Product  Inputs=*/
  Gain : Gain  Gain=100
  Gain1 : Gain  Gain=100
  %H : Outport
  %L : Outport  Port=2
  wires:
  H/1 -> Add/2
  Processo/1 -> Add/1, Divide1/1, Divide2/2, Add1/2
  Divide1/1 -> Gain/1
  Gain/1 -> %H/1
  L/1 -> Add1/1
  Gain1/1 -> %L/1
  Divide2/1 -> Gain1/1
  Add1/1 -> Divide2/1
  Add/1 -> Divide1/2

== system MPC_JUB27_galdir/Subsystem1 ==
  Frequência de Operação : Inport
  PChegada [bar] : Inport  Port=2
  Demux : Demux  Outputs=3
  Mux : Mux  Inputs=2
  S-function1 : S-Function  FunctionName=CalcVazao  Parameters=MatrizSimulador,DeltaT,QIni  SFunctionDeploymentMode=off  EnableBusSupport=off
  Vazão Instantânea (m3/dia) : Outport
  "Óleo Produzido Instantâneo (m3) " : Outport  Port=2
  Óleo Produzido Acumulado (m3) : Outport  Port=3
  wires:
  PChegada [bar]/1 -> Mux/2
  Frequência de Operação/1 -> Mux/1
  Mux/1 -> S-function1/1
  S-function1/1 -> Demux/1
  Demux/2 -> "Óleo Produzido Instantâneo (m3) "/1
  Demux/3 -> Óleo Produzido Acumulado (m3)/1
  Demux/1 -> Vazão Instantânea (m3/dia)/1

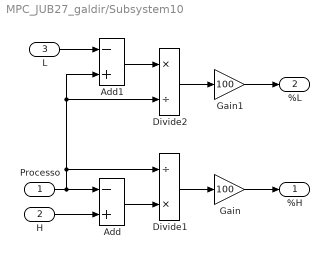
== system MPC_JUB27_galdir/Subsystem10 ==
  Processo : Inport
  H : Inport  Port=2
  L : Inport  Port=3
  Add : Sum  Inputs=-+
  Add1 : Sum  Inputs=-+
  Divide1 : Product  Inputs=/*
  Divide2 : Product  Inputs=*/
  Gain : Gain  Gain=100
  Gain1 : Gain  Gain=100
  %H : Outport
  %L : Outport  Port=2
  wires:
  Add/1 -> Divide1/2
  Add1/1 -> Divide2/1
  Divide2/1 -> Gain1/1
  Gain1/1 -> %L/1
  L/1 -> Add1/1
  Gain/1 -> %H/1
  Divide1/1 -> Gain/1
  Processo/1 -> Add1/2, Divide2/2, Divide1/1, Add/1
  H/1 -> Add/2

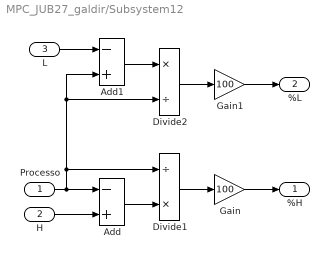
== system MPC_JUB27_galdir/Subsystem12 ==
  Processo : Inport
  H : Inport  Port=2
  L : Inport  Port=3
  Add : Sum  Inputs=-+
  Add1 : Sum  Inputs=-+
  Divide1 : Product  Inputs=/*
  Divide2 : Product  Inputs=*/
  Gain : Gain  Gain=100
  Gain1 : Gain  Gain=100
  %H : Outport
  %L : Outport  Port=2
  wires:
  H/1 -> Add/2
  Processo/1 -> Add/1, Divide1/1, Divide2/2, Add1/2
  Divide1/1 -> Gain/1
  Gain/1 -> %H/1
  L/1 -> Add1/1
  Gain1/1 -> %L/1
  Divide2/1 -> Gain1/1
  Add1/1 -> Divide2/1
  Add/1 -> Divide1/2

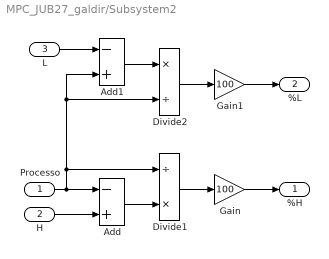
== system MPC_JUB27_galdir/Subsystem2 ==
  Processo : Inport
  H : Inport  Port=2
  L : Inport  Port=3
  Add : Sum  Inputs=-+
  Add1 : Sum  Inputs=-+
  Divide1 : Product  Inputs=/*
  Divide2 : Product  Inputs=*/
  Gain : Gain  Gain=100
  Gain1 : Gain  Gain=100
  %H : Outport
  %L : Outport  Port=2
  wires:
  Add/1 -> Divide1/2
  Add1/1 -> Divide2/1
  Divide2/1 -> Gain1/1
  Gain1/1 -> %L/1
  L/1 -> Add1/1
  Gain/1 -> %H/1
  Divide1/1 -> Gain/1
  Processo/1 -> Add1/2, Divide2/2, Divide1/1, Add/1
  H/1 -> Add/2

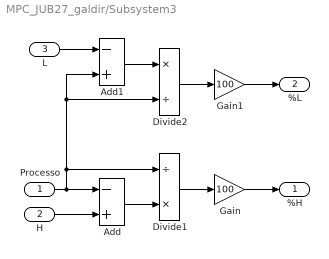
== system MPC_JUB27_galdir/Subsystem3 ==
  Processo : Inport
  H : Inport  Port=2
  L : Inport  Port=3
  Add : Sum  Inputs=-+
  Add1 : Sum  Inputs=-+
  Divide1 : Product  Inputs=/*
  Divide2 : Product  Inputs=*/
  Gain : Gain  Gain=100
  Gain1 : Gain  Gain=100
  %H : Outport
  %L : Outport  Port=2
  wires:
  H/1 -> Add/2
  Processo/1 -> Add/1, Divide1/1, Divide2/2, Add1/2
  Divide1/1 -> Gain/1
  Gain/1 -> %H/1
  L/1 -> Add1/1
  Gain1/1 -> %L/1
  Divide2/1 -> Gain1/1
  Add1/1 -> Divide2/1
  Add/1 -> Divide1/2

== system MPC_JUB27_galdir/Subsystem4 ==
  Processo : Inport
  H : Inport  Port=2
  L : Inport  Port=3
  Add : Sum  Inputs=-+
  Add1 : Sum  Inputs=-+
  Divide1 : Product  Inputs=/*
  Divide2 : Product  Inputs=*/
  Gain : Gain  Gain=100
  Gain1 : Gain  Gain=100
  %H : Outport
  %L : Outport  Port=2
  wires:
  Add/1 -> Divide1/2
  Add1/1 -> Divide2/1
  Divide2/1 -> Gain1/1
  Gain1/1 -> %L/1
  L/1 -> Add1/1
  Gain/1 -> %H/1
  Divide1/1 -> Gain/1
  Processo/1 -> Add1/2, Divide2/2, Divide1/1, Add/1
  H/1 -> Add/2

== system MPC_JUB27_galdir/Subsystem5 ==
  Processo : Inport
  H : Inport  Port=2
  L : Inport  Port=3
  Add : Sum  Inputs=-+
  Add1 : Sum  Inputs=-+
  Divide1 : Product  Inputs=/*
  Divide2 : Product  Inputs=*/
  Gain : Gain  Gain=100
  Gain1 : Gain  Gain=100
  %H : Outport
  %L : Outport  Port=2
  wires:
  H/1 -> Add/2
  Processo/1 -> Add/1, Divide1/1, Divide2/2, Add1/2
  Divide1/1 -> Gain/1
  Gain/1 -> %H/1
  L/1 -> Add1/1
  Gain1/1 -> %L/1
  Divide2/1 -> Gain1/1
  Add1/1 -> Divide2/1
  Add/1 -> Divide1/2

== system MPC_JUB27_galdir/Subsystem6 ==
  Processo : Inport
  H : Inport  Port=2
  L : Inport  Port=3
  Add : Sum  Inputs=-+
  Add1 : Sum  Inputs=-+
  Divide1 : Product  Inputs=/*
  Divide2 : Product  Inputs=*/
  Gain : Gain  Gain=100
  Gain1 : Gain  Gain=100
  %H : Outport
  %L : Outport  Port=2
  wires:
  Add/1 -> Divide1/2
  Add1/1 -> Divide2/1
  Divide2/1 -> Gain1/1
  Gain1/1 -> %L/1
  L/1 -> Add1/1
  Gain/1 -> %H/1
  Divide1/1 -> Gain/1
  Processo/1 -> Add1/2, Divide2/2, Divide1/1, Add/1
  H/1 -> Add/2

== system MPC_JUB27_galdir/Subsystem7 ==
  Processo : Inport
  H : Inport  Port=2
  L : Inport  Port=3
  Add : Sum  Inputs=-+
  Add1 : Sum  Inputs=-+
  Divide1 : Product  Inputs=/*
  Divide2 : Product  Inputs=*/
  Gain : Gain  Gain=100
  Gain1 : Gain  Gain=100
  %H : Outport
  %L : Outport  Port=2
  wires:
  H/1 -> Add/2
  Processo/1 -> Add/1, Divide1/1, Divide2/2, Add1/2
  Divide1/1 -> Gain/1
  Gain/1 -> %H/1
  L/1 -> Add1/1
  Gain1/1 -> %L/1
  Divide2/1 -> Gain1/1
  Add1/1 -> Divide2/1
  Add/1 -> Divide1/2

== system MPC_JUB27_galdir/Subsystem8 ==
  Processo : Inport
  H : Inport  Port=2
  L : Inport  Port=3
  Add : Sum  Inputs=-+
  Add1 : Sum  Inputs=-+
  Divide1 : Product  Inputs=/*
  Divide2 : Product  Inputs=*/
  Gain : Gain  Gain=100
  Gain1 : Gain  Gain=100
  %H : Outport
  %L : Outport  Port=2
  wires:
  Add/1 -> Divide1/2
  Add1/1 -> Divide2/1
  Divide2/1 -> Gain1/1
  Gain1/1 -> %L/1
  L/1 -> Add1/1
  Gain/1 -> %H/1
  Divide1/1 -> Gain/1
  Processo/1 -> Add1/2, Divide2/2, Divide1/1, Add/1
  H/1 -> Add/2

== system MPC_JUB27_galdir/Subsystem9 ==
  Processo : Inport
  H : Inport  Port=2
  L : Inport  Port=3
  Add : Sum  Inputs=-+
  Add1 : Sum  Inputs=-+
  Divide1 : Product  Inputs=/*
  Divide2 : Product  Inputs=*/
  Gain : Gain  Gain=100
  Gain1 : Gain  Gain=100
  %H : Outport
  %L : Outport  Port=2
  wires:
  H/1 -> Add/2
  Processo/1 -> Add/1, Divide1/1, Divide2/2, Add1/2
  Divide1/1 -> Gain/1
  Gain/1 -> %H/1
  L/1 -> Add1/1
  Gain1/1 -> %L/1
  Divide2/1 -> Gain1/1
  Add1/1 -> Divide2/1
  Add/1 -> Divide1/2

== system MPC_JUB27_galdir/Definição de alvos desejados/Plano ENG ==
  Demux : Demux  Outputs=2
  S-Function : S-Function  FunctionName=ExecutaPlano  Parameters=Plano  SFunctionDeploymentMode=off  EnableBusSupport=off
  FreqAlvo [Hz] : Outport
  PMonAlvo [bar] : Outport  Port=2
  wires:
  S-Function/1 -> Demux/1
  Demux/1 -> FreqAlvo [Hz]/1  "Freq"
  Demux/2 -> PMonAlvo [bar]/1  "PMonAlvo"

== system MPC_JUB27_galdir/Definição de alvos desejados/Subsystem13 ==
  Entrada : Inport
  Add : Sum  Inputs=++-
  Delay : Delay  DelayLength=DeltaT/Ts
  Perturbação1 : Step  Time=TIni  After=ValorP  SampleTime=0
  Saida com Perturbação : Outport
  wires:
  Entrada/1 -> Add/2
  Delay/1 -> Add/3
  Add/1 -> Saida com Perturbação/1
  Perturbação1/1 -> Add/1, Delay/1

== system MPC_JUB27_galdir/Definição de alvos desejados/Subsystem14 ==
  Entrada : Inport
  Add : Sum  Inputs=++-
  Delay : Delay  DelayLength=DeltaT/Ts
  Perturbação1 : Step  Time=TIni  After=ValorP  SampleTime=0
  Saida com Perturbação : Outport
  wires:
  Perturbação1/1 -> Delay/1, Add/1
  Add/1 -> Saida com Perturbação/1
  Delay/1 -> Add/3
  Entrada/1 -> Add/2

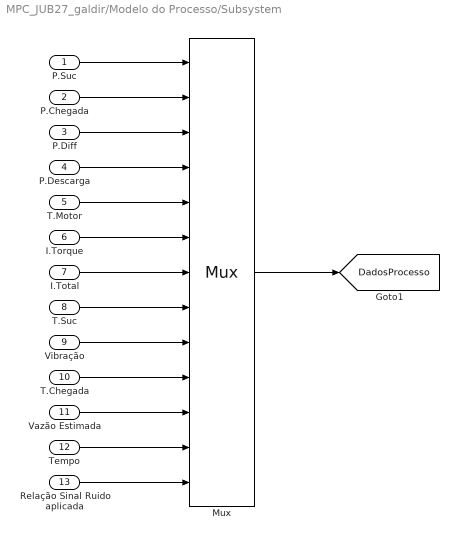
== system MPC_JUB27_galdir/Modelo do Processo/Subsystem ==
  P.Suc : Inport
  P.Chegada : Inport  Port=2
  P.Diff : Inport  Port=3
  P.Descarga : Inport  Port=4
  T.Motor : Inport  Port=5
  I.Torque : Inport  Port=6
  I.Total : Inport  Port=7
  T.Suc : Inport  Port=8
  Vibração : Inport  Port=9
  T.Chegada : Inport  Port=10
  Vazão Estimada : Inport  Port=11
  Tempo : Inport  Port=12
  Relação Sinal Ruido aplicada : Inport  Port=13
  Mux : Mux  Inputs=13
  tag scope: DadosProcesso=global
  wires:
  P.Suc/1 -> Mux/1
  P.Chegada/1 -> Mux/2
  T.Motor/1 -> Mux/5
  I.Torque/1 -> Mux/6
  T.Suc/1 -> Mux/8
  P.Diff/1 -> Mux/3
  I.Total/1 -> Mux/7
  P.Descarga/1 -> Mux/4
  Mux/1 -> [DadosProcesso]
  T.Chegada/1 -> Mux/10
  Vibração/1 -> Mux/9
  Relação Sinal Ruido aplicada/1 -> Mux/13
  Vazão Estimada/1 -> Mux/11
  Tempo/1 -> Mux/12

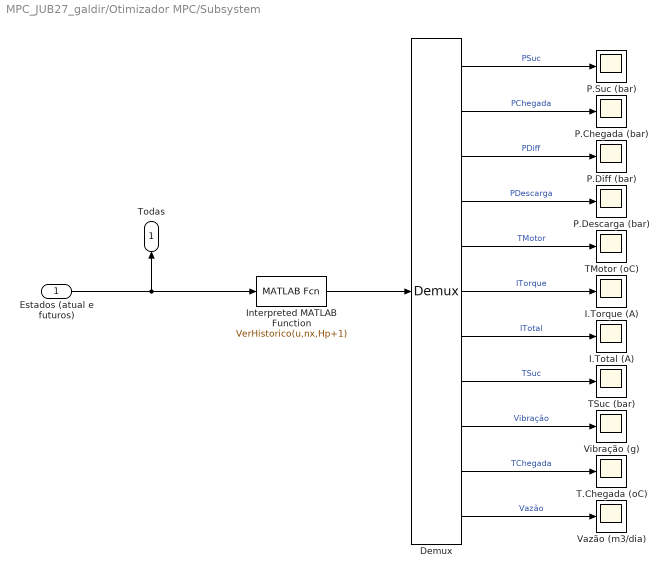
== system MPC_JUB27_galdir/Otimizador MPC/Subsystem ==
  Estados (atual e futuros) : Inport
  Demux : Demux  Outputs=nx
  I.Torque (A) : Scope
  I.Total (A) : Scope
  Interpreted MATLAB Function : MATLABFcn  MATLABFcn=VerHistorico(u,nx,Hp+1)
  P.Chegada (bar) : Scope
  P.Descarga (bar) : Scope
  P.Diff (bar) : Scope
  P.Suc (bar) : Scope
  T.Chegada (oC) : Scope
  TMotor (oC) : Scope
  TSuc (bar) : Scope
  Vazão (m3/dia) : Scope
  Vibração (g) : Scope
  Todas : Outport
  wires:
  Demux/1 -> P.Suc (bar)/1  "PSuc"
  Demux/2 -> P.Chegada (bar)/1  "PChegada"
  Demux/11 -> Vazão (m3/dia)/1  "Vazão"
  Demux/10 -> T.Chegada (oC)/1  "TChegada"
  Demux/9 -> Vibração (g)/1  "Vibração"
  Demux/8 -> TSuc (bar)/1  "TSuc"
  Demux/7 -> I.Total (A)/1  "ITotal"
  Demux/6 -> I.Torque (A)/1  "ITorque"
  Demux/5 -> TMotor (oC)/1  "TMotor"
  Demux/4 -> P.Descarga (bar)/1  "PDescarga"
  Demux/3 -> P.Diff (bar)/1  "PDiff"
  Estados (atual e futuros)/1 -> Interpreted MATLAB Function/1, Todas/1
  Interpreted MATLAB Function/1 -> Demux/1

== system MPC_JUB27_galdir/Otimizador MPC/Subsystem1 ==
  Ações de controle preditas : Inport
  Demux : Demux  Outputs=nu
  Interpreted MATLAB Function : MATLABFcn  MATLABFcn=VerHistorico(u,nu,Hp)
  Scope : Scope
  Scope1 : Scope
  Todas : Outport
  wires:
  Interpreted MATLAB Function/1 -> Demux/1
  Ações de controle preditas/1 -> Todas/1, Interpreted MATLAB Function/1
  Demux/2 -> Scope1/1  "PMonAlvo"
  Demux/1 -> Scope/1  "Freq"
